simulink model "Problem_6"  (R2020a)
settings: Solver=VariableStepAuto  StartTime=0.0  StopTime=10.0  RelTol=1e-3
settings Model: Creator=hp  LastModifiedBy=hp

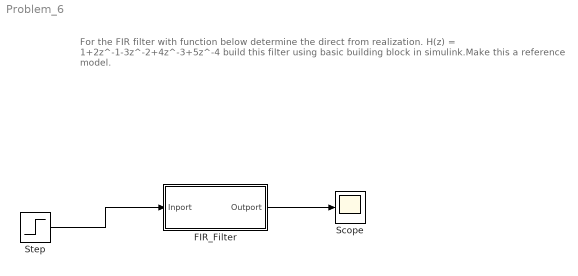
== system Problem_6 ==
  note: For the FIR filter with function below determine the direct from realization.
      | H(z) = 1+2z^-1-3z^-2+4z^-3+5z^-4
      | build this filter using basic building block in simulink.Make this a reference model.
  FIR_Filter : Subsystem
  Scope : Scope
  Step : Step  SampleTime=0
  wires:
  FIR_Filter/1(Outport) -> Scope/1
  Step/1 -> FIR_Filter/1(Inport)

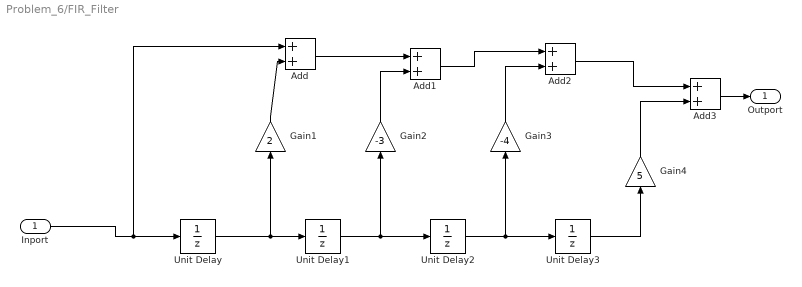
== system Problem_6/FIR_Filter ==
  Inport : Inport
  Add{,1..3} (4 alike) : Sum
  Gain1 : Gain  Gain=2
  Gain2 : Gain  Gain=-3
  Gain3 : Gain  Gain=-4
  Gain4 : Gain  Gain=5
  Unit Delay{,1..3} (4 alike) : UnitDelay  SampleTime=-1  HasFrameUpgradeWarning=on
  Outport : Outport
  wires:
  Add3/1 -> Outport/1
  Unit Delay/1 -> Gain1/1, Unit Delay1/1
  Unit Delay1/1 -> Gain2/1, Unit Delay2/1
  Unit Delay2/1 -> Gain3/1, Unit Delay3/1
  Unit Delay3/1 -> Gain4/1
  Gain4/1 -> Add3/2
  Add2/1 -> Add3/1
  Gain3/1 -> Add2/2
  Gain2/1 -> Add1/2
  Add1/1 -> Add2/1
  Gain1/1 -> Add/2
  Add/1 -> Add1/1
  Inport/1 -> Add/1, Unit Delay/1
